simulink model "Iteration2"  (R2023b)
settings: Solver=VariableStepAuto  StartTime=0.0  StopTime=260  RelTol=1e-3
undefined symbols (not defined in the file): entity, m, n, recordQueueTimeEng1, recordQueueTimeSrEng1, recordQueueTimeSrEng2, recordQueueTimeSrEng3
settings Model: Creator=enos9  LastModifiedBy=enos9
settings SolverCC: AlgebraicLoopSolver=TrustRegion
settings DataIOCC: SaveOutput=off  SaveTime=off
settings DebuggingCC: UnconnectedInputMsg=warning  UnconnectedOutputMsg=warning  UnconnectedLineMsg=warning  ArithmeticOperatorsInVariantConditions=warning
settings ModelReferenceCC: EnableRefExpFcnMdlSchedulingChecks=on
settings SFSimCC: SimUseLocalCustomCode=off  CustomCodeUndefinedFunction=UseInterfaceOnly
settings RTWCC: RTWUseLocalCustomCode=off
settings CodeAppCC: StateflowObjectComments=on

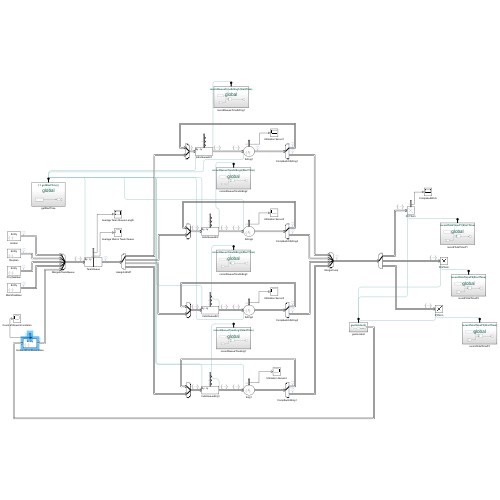
[thumbnail: Simulink's stored preview of the top-level diagram]
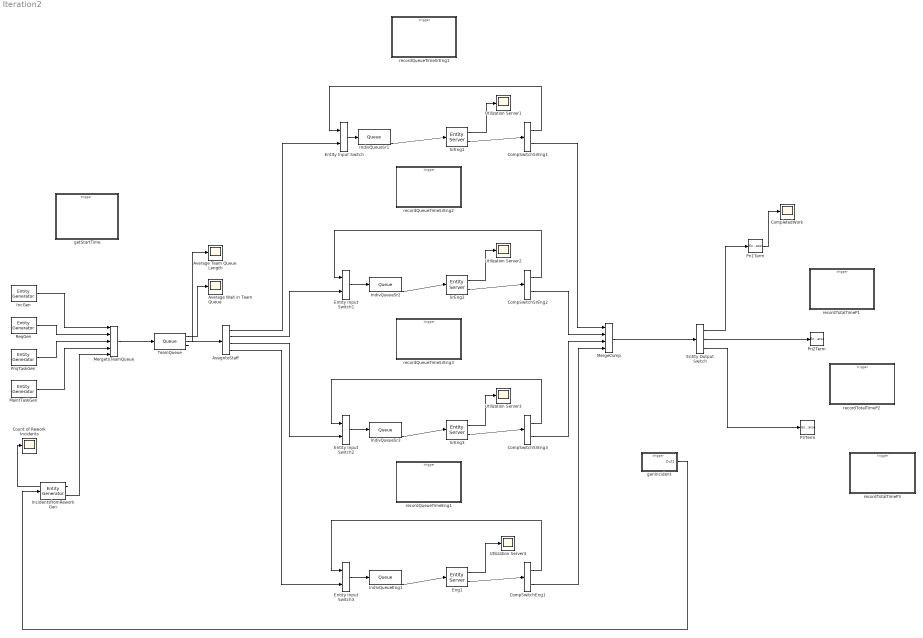
== system Iteration2 ==
  " IndivQueueEng1" : Queue  InputPortMessageModes=m  OutputPortMessageModes=n,n,n,m  Capacity=inf  QueueType=Priority  PrioritySource=Priority  EntryAction=entity.QueueTime = getStartTime();  ExitAction=recordQueueTimeEng1(entity.QueueTime)  NumberEntitiesInBlock=on  AverageWait=on  AverageQueueLength=on
      settings: OutputPortMap=o1,o2,o3,o5
  " IndivQueueSr3" : Queue  InputPortMessageModes=m  OutputPortMessageModes=n,n,n,m  Capacity=inf  QueueType=Priority  PrioritySource=Priority  EntryAction=entity.QueueTime = getStartTime();  ExitAction=recordQueueTimeSrEng3(entity.QueueTime)  NumberEntitiesInBlock=on  AverageWait=on  AverageQueueLength=on
      settings: OutputPortMap=o1,o2,o3,o5
  AssigntoStaff : EntityOutputSwitch  InputPortMessageModes=m  OutputPortMessageModes=m,m,m,m  NumberOutputPorts=4  SwitchingCriterion=Round robin  SwitchAttributeName=Attribute1
      settings: OutputPortMap=o0,o1,o2,o3
  Average Team Queue Length : Scope
  Average Wait in Team Queue : Scope
  CompSwitchEng1 : EntityOutputSwitch  InputPortMessageModes=m  OutputPortMessageModes=m,m  SwitchingCriterion=From attribute  SwitchAttributeName=RemWork
  CompSwitchSrEng1 : EntityOutputSwitch  InputPortMessageModes=m  OutputPortMessageModes=m,m  SwitchingCriterion=From attribute  SwitchAttributeName=RemWork
  CompSwitchSrEng2 : EntityOutputSwitch  InputPortMessageModes=m  OutputPortMessageModes=m,m  SwitchingCriterion=From attribute  SwitchAttributeName=RemWork
  CompSwitchSrEng3 : EntityOutputSwitch  InputPortMessageModes=m  OutputPortMessageModes=m,m  SwitchingCriterion=From attribute  SwitchAttributeName=RemWork
  CompletedWork : Scope
  Count of Rework Incidents : Scope
  Eng1 : EntityServer  InputPortMessageModes=m  OutputPortMessageModes=n,m  Capacity=1  ServiceTimeSource=Attribute  ServiceTimeAttributeName=ReqServiceTime  ServiceTimeAction=|  EntryAction=|  ServiceCompleteAction=|  Utilization=on
      ServiceTimeAction=|
      | mean = .5;
      | dt = -mean*log(1-rand());
      EntryAction=|
      | %entity.ServiceTime = -.3*log(1-rand())         %Base run
      | entity.ServiceTime = -.201*log(1-rand())        %Iteration 2
      | 
      | entity.ServiceStartTime = getStartTime()-entity.QueueTime;
      | 
      | entity.AsignSkillLevel = 2
      | 
      | skilvldiff = entity.AsignSkillLevel - entity.ReqSkillLevel
      | if skilvldiff == 2
      |     entity.ServiceTime = entity.ServiceTime*0.80
      |     entity.Rework = entity.Rework-0.002
      | elseif skilvldiff == 1
      |     entity.ServiceTime = entity.ServiceTime*0.90
      |     entity.Rework = entity.Rework-0.001
      | elseif skilvldiff == -1
      |     entity.ServiceTime = entity.ServiceTime*1.1
      |     entity.Rework = entity.Rework+0.0025
      | elseif skilvldiff == -2
      |     entity.ServiceTime = entity.ServiceTime*1.2
      |     entity.Rework = entity.Rework+0.005
      | end
      ServiceCompleteAction=|
      | svctimediff = entity.ReqServiceTime - entity.ServiceTime
      | 
      | if svctimediff > 0
      |     entity.RemWork = 1
      |     entity.ReqServiceTime = (entity.ReqServiceTime - svctimediff) * 1.1
      | else
      |     entity.RemWork = 2
      | end
      settings: OutputPortMap=o5,o9
  Entity Input Switch : EntityInputSwitch  InputPortMessageModes=m,m  OutputPortMessageModes=m  SwitchingCriterion=Equiprobable
  Entity Input Switch1 : EntityInputSwitch  InputPortMessageModes=m,m  OutputPortMessageModes=m
  Entity Input Switch2 : EntityInputSwitch  InputPortMessageModes=m,m  OutputPortMessageModes=m
  Entity Input Switch3 : EntityInputSwitch  InputPortMessageModes=m,m  OutputPortMessageModes=m
  Entity Output Switch : EntityOutputSwitch  InputPortMessageModes=m  OutputPortMessageModes=m,m,m  NumberOutputPorts=3  SwitchingCriterion=From attribute  SwitchAttributeName=Priority
      settings: OutputPortMap=o0,o1,o2
  IncGen : EntityGenerator  Description=Incident Generator  OutputPortMessageModes=m  TimeSource=MATLAB action  IntergenerationTimeAction=dt = -0.150685*log(1-rand());  GenerateAction=|  AttributeName=Priority|ReqSkillLevel|ReqSkillType|ReqServiceTime|LeadTime|Urgency|RemWork|ServiceTime|AsignSkillLevel|Rework|WorkType|StartTime|QueueTime|ServiceStartTime  AttributeInitialValue=0|0|0|0|0|0|0|0|0|.44|1|1|0|1  EntityType=Structured  EntityTypeName=Entity
      | prnum = rand()                     %Priority
      | 
      | if prnum<0.6
      |     entity.Priority = 3;           %59 percent low priority
      | elseif prnum>0.995
      |     entity.Priority = 1;           %0.5 percent high priority
      | else
      |     entity.Priority = 2            %40.5 percent medium priority
      | end
      | 
      | pslnum = rand()                    %ReqSkillLevel
      | 
      | if pslnum<0.76
      |     entity.ReqSkillLevel = 3;      %75 percent low skill
      | elseif pslnum>0.94
      |     entity.ReqSkillLevel = 1;      %5 percent high skill
      | else
      |     entity.ReqSkillLevel = 2       %20 percent medium skill
      | end
      | 
      | pstnum = rand()                    %ReqSkillType
      | 
      | if pstnum<0.57                    
      |     entity.ReqSkillType = 2;       %56 percent team B (IDM)
      | elseif pstnum>0.89
      |     entity.ReqSkillType = 3;       %10 percent both
      | else
      |     entity.ReqSkillType = 1        %34 percent team A (O365)
      | end
      | 
      | entity.ReqServiceTime = -.2*log(1-rand())       %ReqServiceTime
  IncidentsfromReworkGen : EntityGenerator  InputPortMessageModes=m  OutputPortMessageModes=n,m  GenerationMethod=Event-based  GenerateAction=|  AttributeName=Priority|ReqSkillLevel|ReqSkillType|ReqServiceTime|LeadTime|Urgency|RemWork|ServiceTime|AsignSkillLevel|Rework|WorkType|StartTime|QueueTime|ServiceStartTime  AttributeInitialValue=0|0|0|0|0|0|0|0|0|.44|1|1|0|1  NumberEntitiesDeparted=on  EntityType=Structured  EntityTypeName=Entity
      | prnum = rand()                     %Priority
      | 
      | if prnum<0.6
      |     entity.Priority = 3;           %59 percent low priority
      | elseif prnum>0.995
      |     entity.Priority = 1;           %0.5 percent high priority
      | else
      |     entity.Priority = 2            %40 percent medium priority
      | end
      | 
      | pslnum = rand()                    %ReqSkillLevel
      | 
      | if pslnum<0.76
      |     entity.ReqSkillLevel = 3;      %75 percent low skill
      | elseif pslnum>0.94
      |     entity.ReqSkillLevel = 1;      %5 percent high skill
      | else
      |     entity.ReqSkillLevel = 2       %20 percent medium skill
      | end
      | 
      | pstnum = rand()                    %ReqSkillType
      | 
      | if pstnum<0.57                    
      |     entity.ReqSkillType = 2;       %56 percent team B (IDM)
      | elseif pstnum>0.89
      |     entity.ReqSkillType = 3;       %10 percent both
      | else
      |     entity.ReqSkillType = 1        %34 percent team A (O365)
      | end
      | 
      | entity.ReqServiceTime = -.2*log(1-rand())       %ReqServiceTime
      settings: InputPortMap=u0  OutputPortMap=o0,o3
  IndivQueueSr1 : Queue  InputPortMessageModes=m  OutputPortMessageModes=n,n,n,m  Capacity=inf  QueueType=Priority  PrioritySource=Priority  EntryAction=entity.QueueTime = getStartTime();  ExitAction=recordQueueTimeSrEng1(entity.QueueTime)  NumberEntitiesInBlock=on  AverageWait=on  AverageQueueLength=on
      settings: OutputPortMap=o1,o2,o3,o5
  IndivQueueSr2 : Queue  InputPortMessageModes=m  OutputPortMessageModes=n,n,n,m  Capacity=inf  QueueType=Priority  PrioritySource=Priority  EntryAction=entity.QueueTime = getStartTime();  ExitAction=recordQueueTimeSrEng2(entity.QueueTime)  NumberEntitiesInBlock=on  AverageWait=on  AverageQueueLength=on
      settings: OutputPortMap=o1,o2,o3,o5
  MaintTaskGen : EntityGenerator  Description=Request Generator  OutputPortMessageModes=m  TimeSource=MATLAB action  IntergenerationTimeAction=dt = -1*log(1-rand());  GenerateAction=|  AttributeName=Priority|ReqSkillLevel|ReqSkillType|ReqServiceTime|LeadTime|Urgency|RemWork|ServiceTime|AsignSkillLevel|Rework|WorkType|StartTime|QueueTime|ServiceStartTime  AttributeInitialValue=0|0|0|0|0|0|0|0|0|.44|4|1|0|1  EntityType=Structured  EntityTypeName=Entity
      | prnum = rand()                     %Priority
      | 
      | if prnum<0.6
      |     entity.Priority = 3;           %59 percent low priority
      | elseif prnum>0.995
      |     entity.Priority = 1;           %0.5 percent high priority
      | else
      |     entity.Priority = 2            %40 percent medium priority
      | end
      | 
      | pslnum = rand()                    %ReqSkillLevel
      | 
      | if pslnum<0.76
      |     entity.ReqSkillLevel = 3;      %75 percent low skill
      | elseif pslnum>0.94
      |     entity.ReqSkillLevel = 1;      %5 percent high skill
      | else
      |     entity.ReqSkillLevel = 2       %20 percent medium skill
      | end
      | 
      | pstnum = rand()                    %ReqSkillType
      | 
      | if pstnum<0.57                    
      |     entity.ReqSkillType = 2;       %56 percent team B (IDM)
      | elseif pstnum>0.89
      |     entity.ReqSkillType = 3;       %10 percent both
      | else
      |     entity.ReqSkillType = 1        %34 percent team A (O365)
      | end
      | 
      | entity.ReqServiceTime = -.2*log(1-rand())       %ReqServiceTime
  MergeComp : EntityInputSwitch  InputPortMessageModes=m,m,m,m  OutputPortMessageModes=m  NumberInputPorts=4
      settings: InputPortMap=u1,u2,u3,u4
  MergetoTeamQueue : EntityInputSwitch  InputPortMessageModes=m,m,m,m,m  OutputPortMessageModes=m  NumberInputPorts=5
      settings: InputPortMap=u1,u2,u3,u4,u5
  P3Term : EntityTerminator  InputPortMessageModes=m  EntryAction=|
      | recordTotalTimeP3(entity.StartTime);
      | 
      | rewnum = rand()
      | 
      | if rewnum < entity.Rework
      |     genIncident();
      |     
      | end
  Pri1Term : EntityTerminator  InputPortMessageModes=m  EntryAction=|  NumberEntitiesArrived=on
      | recordTotalTimeP1(entity.StartTime);
      | 
      | rewnum = rand()
      | 
      | if rewnum < entity.Rework
      |     genIncident();
      |     
      | end
      settings: OutputPortMap=o0
  Pri2Term : EntityTerminator  InputPortMessageModes=m  EntryAction=|
      | recordTotalTimeP2(entity.StartTime);
      | 
      | rewnum = rand()
      | 
      | if rewnum < entity.Rework
      |     genIncident();
      |     
      | end
  ProjTaskGen : EntityGenerator  Description=Request Generator  OutputPortMessageModes=m  TimeSource=MATLAB action  IntergenerationTimeAction=dt = -.5*log(1-rand());  GenerateAction=|  AttributeName=Priority|ReqSkillLevel|ReqSkillType|ReqServiceTime|LeadTime|Urgency|RemWork|ServiceTime|AsignSkillLevel|Rework|WorkType|StartTime|QueueTime|ServiceStartTime  AttributeInitialValue=0|0|0|0|0|0|0|0|0|.44|3|1|0|1  EntityType=Structured  EntityTypeName=Entity
      | prnum = rand()                     %Priority
      | 
      | if prnum<0.6
      |     entity.Priority = 3;           %59 percent low priority
      | elseif prnum>0.995
      |     entity.Priority = 1;           %0.5 percent high priority
      | else
      |     entity.Priority = 2            %40 percent medium priority
      | end
      | 
      | pslnum = rand()                    %ReqSkillLevel
      | 
      | if pslnum<0.76
      |     entity.ReqSkillLevel = 3;      %75 percent low skill
      | elseif pslnum>0.94
      |     entity.ReqSkillLevel = 1;      %5 percent high skill
      | else
      |     entity.ReqSkillLevel = 2       %20 percent medium skill
      | end
      | 
      | pstnum = rand()                    %ReqSkillType
      | 
      | if pstnum<0.57                    
      |     entity.ReqSkillType = 2;       %56 percent team B (IDM)
      | elseif pstnum>0.89
      |     entity.ReqSkillType = 3;       %10 percent both
      | else
      |     entity.ReqSkillType = 1        %34 percent team A (O365)
      | end
      | 
      | entity.ReqServiceTime = -.2*log(1-rand())       %ReqServiceTime
  ReqGen : EntityGenerator  Description=Request Generator  OutputPortMessageModes=m  TimeSource=MATLAB action  IntergenerationTimeAction=dt = -0.061303*log(1-rand());  GenerateAction=|  AttributeName=Priority|ReqSkillLevel|ReqSkillType|ReqServiceTime|LeadTime|Urgency|RemWork|ServiceTime|AsignSkillLevel|Rework|WorkType|StartTime|QueueTime|ServiceStartTime  AttributeInitialValue=0|0|0|0|0|0|0|0|0|.44|2|1|0|1  EntityType=Structured  EntityTypeName=Entity
      | prnum = rand()                     %Priority
      | 
      | if prnum<0.6
      |     entity.Priority = 3;           %59 percent low priority
      | elseif prnum>0.995
      |     entity.Priority = 1;           %0.5 percent high priority
      | else
      |     entity.Priority = 2            %40 percent medium priority
      | end
      | 
      | pslnum = rand()                    %ReqSkillLevel
      | 
      | if pslnum<0.76
      |     entity.ReqSkillLevel = 3;      %75 percent low skill
      | elseif pslnum>0.94
      |     entity.ReqSkillLevel = 1;      %5 percent high skill
      | else
      |     entity.ReqSkillLevel = 2       %20 percent medium skill
      | end
      | 
      | pstnum = rand()                    %ReqSkillType
      | 
      | if pstnum<0.57                    
      |     entity.ReqSkillType = 2;       %56 percent team B (IDM)
      | elseif pstnum>0.89
      |     entity.ReqSkillType = 3;       %10 percent both
      | else
      |     entity.ReqSkillType = 1        %34 percent team A (O365)
      | end
      | 
      | entity.ReqServiceTime = -.2*log(1-rand())       %ReqServiceTime
  SrEng1 : EntityServer  InputPortMessageModes=m  OutputPortMessageModes=n,m  Capacity=1  ServiceTimeSource=Attribute  ServiceTimeAttributeName=ReqServiceTime  ServiceTimeAction=|  EntryAction=|  ServiceCompleteAction=|  Utilization=on
      ServiceTimeAction=|
      | mean = .3;
      | dt = -mean*log(1-rand());
      EntryAction=|
      | %entity.ServiceTime = -.3*log(1-rand())         %Base run
      | entity.ServiceTime = -.201*log(1-rand())        %Iteration 2
      | 
      | entity.ServiceStartTime = getStartTime()-entity.QueueTime;
      | 
      | entity.AsignSkillLevel = 1
      | 
      | skilvldiff = entity.AsignSkillLevel - entity.ReqSkillLevel
      | if skilvldiff == 2
      |     entity.ServiceTime = entity.ServiceTime*0.80
      |     entity.Rework = entity.Rework-0.002
      | elseif skilvldiff == 1
      |     entity.ServiceTime = entity.ServiceTime*0.90
      |     entity.Rework = entity.Rework-0.001
      | elseif skilvldiff == -1
      |     entity.ServiceTime = entity.ServiceTime*1.1
      |     entity.Rework = entity.Rework+0.0025
      | elseif skilvldiff == -2
      |     entity.ServiceTime = entity.ServiceTime*1.2
      |     entity.Rework = entity.Rework+0.005
      | end
      ServiceCompleteAction=|
      | svctimediff = entity.ReqServiceTime - entity.ServiceTime
      | 
      | if svctimediff > 0
      |     entity.RemWork = 1
      |     entity.ReqServiceTime = (entity.ReqServiceTime - svctimediff) * 1.1
      | else
      |     entity.RemWork = 2
      | end
      settings: OutputPortMap=o5,o9
  SrEng2 : EntityServer  InputPortMessageModes=m  OutputPortMessageModes=n,m  Capacity=1  ServiceTimeSource=Attribute  ServiceTimeAttributeName=ReqServiceTime  ServiceTimeAction=|  EntryAction=|  ServiceCompleteAction=|  Utilization=on
      ServiceTimeAction=|
      | mean = .3;
      | dt = -mean*log(1-rand());
      EntryAction=|
      | %entity.ServiceTime = -.3*log(1-rand())         %Base run
      | entity.ServiceTime = -.201*log(1-rand())        %Iteration 2
      | 
      | entity.ServiceStartTime = getStartTime()-entity.QueueTime;
      | 
      | entity.AsignSkillLevel = 1
      | 
      | skilvldiff = entity.AsignSkillLevel - entity.ReqSkillLevel
      | if skilvldiff == 2
      |     entity.ServiceTime = entity.ServiceTime*0.80
      |     entity.Rework = entity.Rework-0.002
      | elseif skilvldiff == 1
      |     entity.ServiceTime = entity.ServiceTime*0.90
      |     entity.Rework = entity.Rework-0.001
      | elseif skilvldiff == -1
      |     entity.ServiceTime = entity.ServiceTime*1.1
      |     entity.Rework = entity.Rework+0.0025
      | elseif skilvldiff == -2
      |     entity.ServiceTime = entity.ServiceTime*1.2
      |     entity.Rework = entity.Rework+0.005
      | end
      ServiceCompleteAction=|
      | svctimediff = entity.ReqServiceTime - entity.ServiceTime
      | 
      | if svctimediff > 0
      |     entity.RemWork = 1
      |     entity.ReqServiceTime = (entity.ReqServiceTime - svctimediff) * 1.1
      | else
      |     entity.RemWork = 2
      | end
      settings: OutputPortMap=o5,o9
  SrEng3 : EntityServer  InputPortMessageModes=m  OutputPortMessageModes=n,m  Capacity=1  ServiceTimeSource=Attribute  ServiceTimeAttributeName=ReqServiceTime  ServiceTimeAction=|  EntryAction=|  ServiceCompleteAction=|  Utilization=on
      ServiceTimeAction=|
      | mean = .3;
      | dt = -mean*log(1-rand());
      EntryAction=|
      | %entity.ServiceTime = -.3*log(1-rand())         %Base run
      | entity.ServiceTime = -.201*log(1-rand())        %Iteration 2
      | 
      | entity.ServiceStartTime = getStartTime()-entity.QueueTime;
      | 
      | entity.AsignSkillLevel = 1
      | 
      | skilvldiff = entity.AsignSkillLevel - entity.ReqSkillLevel
      | if skilvldiff == 2
      |     entity.ServiceTime = entity.ServiceTime*0.80
      |     entity.Rework = entity.Rework-0.002
      | elseif skilvldiff == 1
      |     entity.ServiceTime = entity.ServiceTime*0.90
      |     entity.Rework = entity.Rework-0.001
      | elseif skilvldiff == -1
      |     entity.ServiceTime = entity.ServiceTime*1.1
      |     entity.Rework = entity.Rework+0.0025
      | elseif skilvldiff == -2
      |     entity.ServiceTime = entity.ServiceTime*1.2
      |     entity.Rework = entity.Rework+0.005
      | end
      ServiceCompleteAction=|
      | svctimediff = entity.ReqServiceTime - entity.ServiceTime
      | 
      | if svctimediff > 0
      |     entity.RemWork = 1
      |     entity.ReqServiceTime = (entity.ReqServiceTime - svctimediff) * 1.1
      | else
      |     entity.RemWork = 2
      | end
      settings: OutputPortMap=o5,o9
  TeamQueue : Queue  Description=Team Queue  InputPortMessageModes=m  OutputPortMessageModes=n,n,m  Capacity=inf  QueueType=Priority  PrioritySource=Priority  EntryAction=entity.StartTime = getStartTime();  AverageWait=on  AverageQueueLength=on
      settings: OutputPortMap=o2,o3,o5
  Utilization Server{1..4} (4 alike) : Scope
  genIncident : Subsystem  TreatAsAtomicUnit=on
  getStartTime : Subsystem  TreatAsAtomicUnit=on
  recordQueueTimeEng1 : Subsystem  TreatAsAtomicUnit=on
  recordQueueTimeSrEng1 : Subsystem  TreatAsAtomicUnit=on
  recordQueueTimeSrEng2 : Subsystem  TreatAsAtomicUnit=on
  recordQueueTimeSrEng3 : Subsystem  TreatAsAtomicUnit=on
  recordTotalTimeP1 : Subsystem  TreatAsAtomicUnit=on
  recordTotalTimeP2 : Subsystem  TreatAsAtomicUnit=on
  recordTotalTimeP3 : Subsystem  TreatAsAtomicUnit=on
  wires:
  IndivQueueSr1/4 -> SrEng1/1
  SrEng1/2 -> CompSwitchSrEng1/1
  IncGen/1 -> MergetoTeamQueue/1
  ReqGen/1 -> MergetoTeamQueue/2
  TeamQueue/3 -> AssigntoStaff/1
  SrEng2/2 -> CompSwitchSrEng2/1
  IndivQueueSr2/4 -> SrEng2/1
  AssigntoStaff/1 -> Entity Input Switch/2
  AssigntoStaff/2 -> Entity Input Switch1/2
  SrEng3/2 -> CompSwitchSrEng3/1
  " IndivQueueSr3"/4 -> SrEng3/1
  AssigntoStaff/3 -> Entity Input Switch2/2
  Eng1/2 -> CompSwitchEng1/1
  " IndivQueueEng1"/4 -> Eng1/1
  AssigntoStaff/4 -> Entity Input Switch3/2
  TeamQueue/2 -> Average Team Queue Length/1
  SrEng1/1 -> Utilization Server1/1
  SrEng2/1 -> Utilization Server2/1
  SrEng3/1 -> Utilization Server3/1
  Eng1/1 -> Utilization Server4/1
  ProjTaskGen/1 -> MergetoTeamQueue/3
  MergeComp/1 -> Entity Output Switch/1
  TeamQueue/1 -> Average Wait in Team Queue/1
  MaintTaskGen/1 -> MergetoTeamQueue/4
  MergetoTeamQueue/1 -> TeamQueue/1
  CompSwitchSrEng1/1 -> Entity Input Switch/1
  Entity Input Switch/1 -> IndivQueueSr1/1
  CompSwitchSrEng1/2 -> MergeComp/1
  CompSwitchSrEng2/2 -> MergeComp/2
  CompSwitchSrEng2/1 -> Entity Input Switch1/1
  Entity Input Switch1/1 -> IndivQueueSr2/1
  CompSwitchSrEng3/1 -> Entity Input Switch2/1
  CompSwitchSrEng3/2 -> MergeComp/3
  Entity Input Switch2/1 -> " IndivQueueSr3"/1
  CompSwitchEng1/1 -> Entity Input Switch3/1
  Entity Input Switch3/1 -> " IndivQueueEng1"/1
  CompSwitchEng1/2 -> MergeComp/4
  IncidentsfromReworkGen/2 -> MergetoTeamQueue/5
  genIncident/1(Out1) -> IncidentsfromReworkGen/1
  IncidentsfromReworkGen/1 -> Count of Rework Incidents/1
  Pri1Term/1 -> CompletedWork/1
  Entity Output Switch/1 -> Pri1Term/1
  Entity Output Switch/2 -> Pri2Term/1
  Entity Output Switch/3 -> P3Term/1

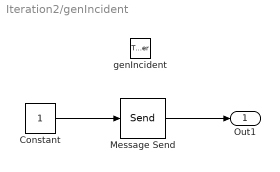
== system Iteration2/genIncident ==
  genIncident : TriggerPort  TriggerType=function-call  IsSimulinkFunction=on  FunctionName=genIncident  FunctionVisibility=scoped  VariantControl=(inherit)
  Constant : Constant
  Message Send : Send  OutputPortMessageModes=m
  Out1 : Outport
  wires:
  Constant/1 -> Message Send/1
  Message Send/1 -> Out1/1

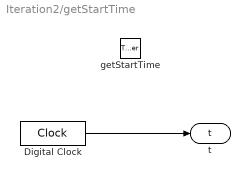
== system Iteration2/getStartTime ==
  getStartTime : TriggerPort  TriggerType=function-call  IsSimulinkFunction=on  FunctionName=getStartTime  VariantControl=(inherit)
  Digital Clock : DigitalClock  SampleTime=-1
  t : ArgOut  DisableCoverage=on  ArgumentName=t
  wires:
  Digital Clock/1 -> t/1

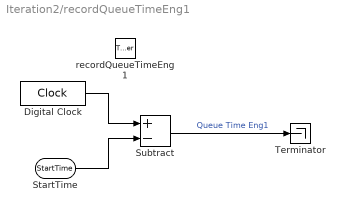
== system Iteration2/recordQueueTimeEng1 ==
  recordQueueTimeEng1 : TriggerPort  TriggerType=function-call  IsSimulinkFunction=on  FunctionName=recordQueueTimeEng1  VariantControl=(inherit)
  Digital Clock : DigitalClock  SampleTime=-1
  Subtract : Sum  Inputs=+-
  Terminator : Terminator
  StartTime : ArgIn  DisableCoverage=on  ArgumentName=StartTime
  wires:
  StartTime/1 -> Subtract/2
  Digital Clock/1 -> Subtract/1
  Subtract/1 -> Terminator/1  "Queue Time Eng1"

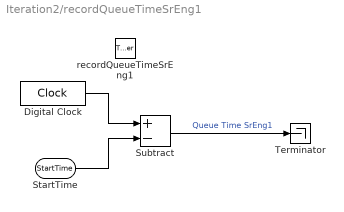
== system Iteration2/recordQueueTimeSrEng1 ==
  recordQueueTimeSrEng1 : TriggerPort  TriggerType=function-call  IsSimulinkFunction=on  FunctionName=recordQueueTimeSrEng1  VariantControl=(inherit)
  Digital Clock : DigitalClock  SampleTime=-1
  Subtract : Sum  Inputs=+-
  Terminator : Terminator
  StartTime : ArgIn  DisableCoverage=on  ArgumentName=StartTime
  wires:
  StartTime/1 -> Subtract/2
  Digital Clock/1 -> Subtract/1
  Subtract/1 -> Terminator/1  "Queue Time SrEng1"

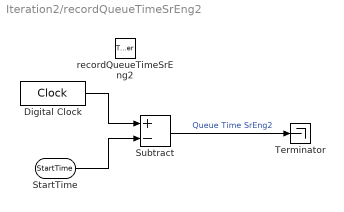
== system Iteration2/recordQueueTimeSrEng2 ==
  recordQueueTimeSrEng2 : TriggerPort  TriggerType=function-call  IsSimulinkFunction=on  FunctionName=recordQueueTimeSrEng2  VariantControl=(inherit)
  Digital Clock : DigitalClock  SampleTime=-1
  Subtract : Sum  Inputs=+-
  Terminator : Terminator
  StartTime : ArgIn  DisableCoverage=on  ArgumentName=StartTime
  wires:
  StartTime/1 -> Subtract/2
  Digital Clock/1 -> Subtract/1
  Subtract/1 -> Terminator/1  "Queue Time SrEng2"

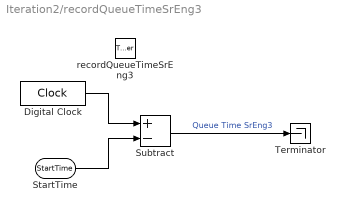
== system Iteration2/recordQueueTimeSrEng3 ==
  recordQueueTimeSrEng3 : TriggerPort  TriggerType=function-call  IsSimulinkFunction=on  FunctionName=recordQueueTimeSrEng3  VariantControl=(inherit)
  Digital Clock : DigitalClock  SampleTime=-1
  Subtract : Sum  Inputs=+-
  Terminator : Terminator
  StartTime : ArgIn  DisableCoverage=on  ArgumentName=StartTime
  wires:
  StartTime/1 -> Subtract/2
  Digital Clock/1 -> Subtract/1
  Subtract/1 -> Terminator/1  "Queue Time SrEng3"

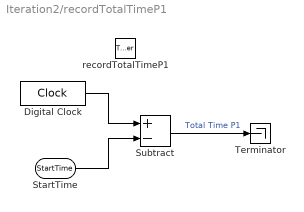
== system Iteration2/recordTotalTimeP1 ==
  recordTotalTimeP1 : TriggerPort  TriggerType=function-call  IsSimulinkFunction=on  FunctionName=recordTotalTimeP1  VariantControl=(inherit)
  Digital Clock : DigitalClock  SampleTime=-1
  Subtract : Sum  Inputs=+-
  Terminator : Terminator
  StartTime : ArgIn  DisableCoverage=on  ArgumentName=StartTime
  wires:
  StartTime/1 -> Subtract/2
  Digital Clock/1 -> Subtract/1
  Subtract/1 -> Terminator/1  "Total Time P1"

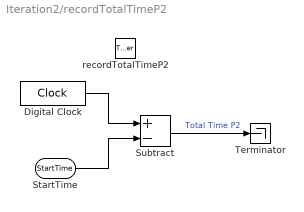
== system Iteration2/recordTotalTimeP2 ==
  recordTotalTimeP2 : TriggerPort  TriggerType=function-call  IsSimulinkFunction=on  FunctionName=recordTotalTimeP2  VariantControl=(inherit)
  Digital Clock : DigitalClock  SampleTime=-1
  Subtract : Sum  Inputs=+-
  Terminator : Terminator
  StartTime : ArgIn  DisableCoverage=on  ArgumentName=StartTime
  wires:
  StartTime/1 -> Subtract/2
  Digital Clock/1 -> Subtract/1
  Subtract/1 -> Terminator/1  "Total Time P2"

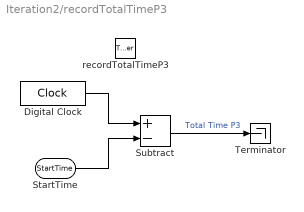
== system Iteration2/recordTotalTimeP3 ==
  recordTotalTimeP3 : TriggerPort  TriggerType=function-call  IsSimulinkFunction=on  FunctionName=recordTotalTimeP3  VariantControl=(inherit)
  Digital Clock : DigitalClock  SampleTime=-1
  Subtract : Sum  Inputs=+-
  Terminator : Terminator
  StartTime : ArgIn  DisableCoverage=on  ArgumentName=StartTime
  wires:
  StartTime/1 -> Subtract/2
  Digital Clock/1 -> Subtract/1
  Subtract/1 -> Terminator/1  "Total Time P3"
